simulink model "DFADAS2_SenFus_v1_201204RC_training_210115"  (R2018b)
settings: Solver=FixedStepDiscrete  StartTime=0.0  StopTime=inf  FixedStep=0.002  RelTol=1e-3  EnableMultiTasking=on
PreLoadFcn:
  | RTWConfigurationCB('preloadfcn', bdroot);
libraries: canmsglib x108, simulink x48, canfdmsglib x12
(part 15 of 28)

== system DFADAS2_SenFus_v1_201204RC_training_210115/Signal Input (Input)/Signal Input (50ms) (Input50)/Front Right Radar(S3) Objects Information (FRRdr)/S0 Data Frame Read/Enabled Subsystem/M2ObjInfo ==
  msg : Inport
  MValue : Inport  Port=2
  RemainderCnt : Inport  Port=3
  obj_num : Inport  Port=4
  Add3 : Sum
  Bus Creator1 : BusCreator  Inputs=24
  Bus Creator2 : BusCreator  Inputs=24
  Constant : Constant  Value=5
  Data Type Conversion{,1..3} (4 alike) : DataTypeConversion  OutDataTypeStr=uint16
  Data Type Conversion5 : DataTypeConversion  OutDataTypeStr=int16
  Demux : Demux  Outputs=24
  Demux1 : Demux  Outputs=24
  If : If  NumInputs=3  IfExpression=u1 == 1  ElseIfExpressions=u2 == 0 & u3 == 1  ShowElse=off
  If Action Subsystem1 : Subsystem  TreatAsAtomicUnit=on
  If Action Subsystem2 : Subsystem  TreatAsAtomicUnit=on
  MValueSel : Constant  Value=2
  Memory1 : Memory  InheritSampleTime=on
  Memory3 : Memory  InheritSampleTime=on
  Merge : Merge
  Merge1 : Merge
  Relational Operator : RelationalOperator  Operator===  OutDataTypeStr=boolean  RndMeth=Simplest
  Relational Operator1 : RelationalOperator  Operator=>  OutDataTypeStr=boolean  RndMeth=Simplest
  Subsystem1 : Subsystem
  Subtract : Sum  Inputs=+-
  M20ObjInfo : Outport
  M21ObjInfo : Outport  Port=2
  wires:
  msg/1 -> If Action Subsystem1/1(msg)
  MValue/1 -> Relational Operator/2
  Subsystem1/1(Out) -> Add3/2
  Add3/1 -> Memory3/1, Data Type Conversion2/1  "MValueSim"
  Data Type Conversion/1 -> Add3/1
  If/1 -> If Action Subsystem1/Action
  If/2 -> If Action Subsystem2/Action
  Relational Operator/1 -> Data Type Conversion/1, Data Type Conversion1/1
  If Action Subsystem1/1(M20ObjInfo) -> Merge/1
  If Action Subsystem2/1(ZeroObjInfo0) -> Merge/2
  MValueSel/1 -> If Action Subsystem1/2("MValueSel "), Relational Operator/1
  If Action Subsystem2/2(ZeroObjInfo1) -> Merge1/2
  If Action Subsystem1/2(M21ObjInfo) -> Merge1/1
  Data Type Conversion1/1 -> If/1
  Data Type Conversion2/1 -> If/2
  Data Type Conversion3/1 -> If/3
  Merge/1 -> Demux/1
  Bus Creator1/1 -> M20ObjInfo/1  "Obj5Info"
  Demux/24 -> Bus Creator1/24  "YVelocityStd_S0_005"
  Demux/10 -> Bus Creator1/10  "Width_S0_005"
  Demux/13 -> Bus Creator1/13  "ExistenceProb_S0_005"
  Demux/17 -> Bus Creator1/17  "ReferencePoint_S0_005"
  Demux/22 -> Bus Creator1/22  "YAccStd_S0_005"
  Demux/7 -> Bus Creator1/7  "YVelocity_S0_005"
  Demux/20 -> Bus Creator1/20  "XPosStd_S0_005"
  Demux/18 -> Bus Creator1/18  "Height_S0_005"
  Demux/12 -> Bus Creator1/12  "Orientation_S0_005"
  Demux/9 -> Bus Creator1/9  "YAcc_S0_005"
  Demux/14 -> Bus Creator1/14  "MovingState_S0_005"
  Demux/5 -> Bus Creator1/5  "YPos_S0_005"
  Demux/23 -> Bus Creator1/23  "YPosStd_S0_005"
  Demux/3 -> Bus Creator1/3  "ObjMeasured_S0_005"
  Demux/16 -> Bus Creator1/16  "ClassHighestProb_S0_005"
  Demux/21 -> Bus Creator1/21  "XVelocityStd_S0_005"
  Demux/4 -> Bus Creator1/4  "XPos_S0_005"
  Demux/19 -> Bus Creator1/19  "XAccStd_S0_005"
  Demux/8 -> Bus Creator1/8  "XAcc_S0_005"
  Demux/2 -> Bus Creator1/2  "ObjInit_S0_005"
  Demux/11 -> Bus Creator1/11  "Length_S0_005"
  Demux/15 -> Bus Creator1/15  "ClassHighest_S0_005"
  Demux/1 -> Bus Creator1/1  "Id_S0_005"
  Demux/6 -> Bus Creator1/6  "XVelocity_S0_005"
  Demux1/1 -> Bus Creator2/1  "Id_S0_006"
  Demux1/6 -> Bus Creator2/6  "XVelocity_S0_006"
  Demux1/2 -> Bus Creator2/2  "ObjInit_S0_006"
  Demux1/3 -> Bus Creator2/3  "ObjMeasured_S0_006"
  Demux1/5 -> Bus Creator2/5  "YPos_S0_006"
  Demux1/16 -> Bus Creator2/16  "ClassHighestProb_S0_006"
  Demux1/4 -> Bus Creator2/4  "XPos_S0_006"
  Demux1/10 -> Bus Creator2/10  "Width_S0_006"
  Demux1/11 -> Bus Creator2/11  "Length_S0_006"
  Demux1/24 -> Bus Creator2/24  "YVelocityStd_S0_006"
  Demux1/9 -> Bus Creator2/9  "YAcc_S0_006"
  Demux1/13 -> Bus Creator2/13  "ExistenceProb_S0_006"
  Demux1/20 -> Bus Creator2/20  "XPosStd_S0_006"
  Demux1/14 -> Bus Creator2/14  "MovingState_S0_006"
  Demux1/7 -> Bus Creator2/7  "YVelocity_S0_006"
  Demux1/15 -> Bus Creator2/15  "ClassHighest_S0_006"
  Demux1/18 -> Bus Creator2/18  "Height_S0_006"
  Demux1/19 -> Bus Creator2/19  "XAccStd_S0_006"
  Demux1/21 -> Bus Creator2/21  "XVelocityStd_S0_006"
  Demux1/8 -> Bus Creator2/8  "XAcc_S0_006"
  Demux1/23 -> Bus Creator2/23  "YPosStd_S0_006"
  Demux1/22 -> Bus Creator2/22  "YAccStd_S0_006"
  Demux1/17 -> Bus Creator2/17  "ReferencePoint_S0_006"
  Demux1/12 -> Bus Creator2/12  "Orientation_S0_006"
  Merge1/1 -> Demux1/1
  Bus Creator2/1 -> M21ObjInfo/1  "Obj6Info"
  Relational Operator1/1 -> If Action Subsystem1/3("obj_count_trorfa ")
  Constant/1 -> Relational Operator1/2
  obj_num/1 -> Relational Operator1/1
  Subtract/1 -> Subsystem1/1(const)
  RemainderCnt/1 -> Data Type Conversion5/1, Data Type Conversion3/1
  Memory1/1 -> Subtract/2
  Data Type Conversion5/1 -> Subtract/1, Memory1/1
  Memory3/1 -> Subsystem1/3(In)

== system DFADAS2_SenFus_v1_201204RC_training_210115/Signal Input (Input)/Signal Input (50ms) (Input50)/Front Right Radar(S3) Objects Information (FRRdr)/S0 Data Frame Read/Enabled Subsystem/M3ObjInfo ==
  msg : Inport
  MValue : Inport  Port=2
  RemainderCnt : Inport  Port=3
  obj_num : Inport  Port=4
  Add3 : Sum
  Bus Creator1 : BusCreator  Inputs=24
  Bus Creator2 : BusCreator  Inputs=24
  Constant : Constant  Value=7
  Data Type Conversion{,1..3} (4 alike) : DataTypeConversion  OutDataTypeStr=uint16
  Data Type Conversion5 : DataTypeConversion  OutDataTypeStr=int16
  Demux : Demux  Outputs=24
  Demux1 : Demux  Outputs=24
  If : If  NumInputs=3  IfExpression=u1 == 1  ElseIfExpressions=u2 == 0 & u3 == 1  ShowElse=off
  If Action Subsystem1 : Subsystem  TreatAsAtomicUnit=on
  If Action Subsystem2 : Subsystem  TreatAsAtomicUnit=on
  MValueSel : Constant  Value=3
  Memory1 : Memory  InheritSampleTime=on
  Memory3 : Memory  InheritSampleTime=on
  Merge : Merge
  Merge1 : Merge
  Relational Operator : RelationalOperator  Operator===  OutDataTypeStr=boolean  RndMeth=Simplest
  Relational Operator1 : RelationalOperator  Operator=>  OutDataTypeStr=boolean  RndMeth=Simplest
  Subsystem1 : Subsystem
  Subtract : Sum  Inputs=+-
  M30ObjInfo : Outport
  M31ObjInfo : Outport  Port=2
  wires:
  Bus Creator2/1 -> M31ObjInfo/1  "Obj8Info"
  Merge1/1 -> Demux1/1
  Demux1/12 -> Bus Creator2/12  "Orientation_S0_008"
  Demux1/17 -> Bus Creator2/17  "ReferencePoint_S0_008"
  Demux1/22 -> Bus Creator2/22  "YAccStd_S0_008"
  Demux1/23 -> Bus Creator2/23  "YPosStd_S0_008"
  Demux1/8 -> Bus Creator2/8  "XAcc_S0_008"
  Demux1/21 -> Bus Creator2/21  "XVelocityStd_S0_008"
  Demux1/19 -> Bus Creator2/19  "XAccStd_S0_008"
  Demux1/18 -> Bus Creator2/18  "Height_S0_008"
  Demux1/15 -> Bus Creator2/15  "ClassHighest_S0_008"
  Demux1/7 -> Bus Creator2/7  "YVelocity_S0_008"
  Demux1/14 -> Bus Creator2/14  "MovingState_S0_008"
  Demux1/20 -> Bus Creator2/20  "XPosStd_S0_008"
  Demux1/13 -> Bus Creator2/13  "ExistenceProb_S0_008"
  Demux1/9 -> Bus Creator2/9  "YAcc_S0_008"
  Demux1/24 -> Bus Creator2/24  "YVelocityStd_S0_008"
  Demux1/11 -> Bus Creator2/11  "Length_S0_008"
  Demux1/10 -> Bus Creator2/10  "Width_S0_008"
  Demux1/4 -> Bus Creator2/4  "XPos_S0_008"
  Demux1/16 -> Bus Creator2/16  "ClassHighestProb_S0_008"
  Demux1/5 -> Bus Creator2/5  "YPos_S0_008"
  Demux1/3 -> Bus Creator2/3  "ObjMeasured_S0_008"
  Demux1/2 -> Bus Creator2/2  "ObjInit_S0_008"
  Demux1/6 -> Bus Creator2/6  "XVelocity_S0_008"
  Demux1/1 -> Bus Creator2/1  "Id_S0_008"
  Demux/6 -> Bus Creator1/6  "XVelocity_S0_007"
  Demux/1 -> Bus Creator1/1  "Id_S0_007"
  Demux/15 -> Bus Creator1/15  "ClassHighest_S0_007"
  Demux/11 -> Bus Creator1/11  "Length_S0_007"
  Demux/2 -> Bus Creator1/2  "ObjInit_S0_007"
  Demux/8 -> Bus Creator1/8  "XAcc_S0_007"
  Demux/19 -> Bus Creator1/19  "XAccStd_S0_007"
  Demux/4 -> Bus Creator1/4  "XPos_S0_007"
  Demux/21 -> Bus Creator1/21  "XVelocityStd_S0_007"
  Demux/16 -> Bus Creator1/16  "ClassHighestProb_S0_007"
  Demux/3 -> Bus Creator1/3  "ObjMeasured_S0_007"
  Demux/23 -> Bus Creator1/23  "YPosStd_S0_007"
  Demux/5 -> Bus Creator1/5  "YPos_S0_007"
  Demux/14 -> Bus Creator1/14  "MovingState_S0_007"
  Demux/9 -> Bus Creator1/9  "YAcc_S0_007"
  Demux/12 -> Bus Creator1/12  "Orientation_S0_007"
  Demux/18 -> Bus Creator1/18  "Height_S0_007"
  Demux/20 -> Bus Creator1/20  "XPosStd_S0_007"
  Demux/7 -> Bus Creator1/7  "YVelocity_S0_007"
  Demux/22 -> Bus Creator1/22  "YAccStd_S0_007"
  Demux/17 -> Bus Creator1/17  "ReferencePoint_S0_007"
  Demux/13 -> Bus Creator1/13  "ExistenceProb_S0_007"
  Demux/10 -> Bus Creator1/10  "Width_S0_007"
  Demux/24 -> Bus Creator1/24  "YVelocityStd_S0_007"
  Bus Creator1/1 -> M30ObjInfo/1  "Obj7Info"
  Merge/1 -> Demux/1
  Data Type Conversion3/1 -> If/3
  Data Type Conversion2/1 -> If/2
  Data Type Conversion1/1 -> If/1
  If Action Subsystem1/2(M31ObjInfo) -> Merge1/1
  If Action Subsystem2/2(ZeroObjInfo1) -> Merge1/2
  MValueSel/1 -> Relational Operator/1, If Action Subsystem1/2("MValueSel ")
  If Action Subsystem2/1(ZeroObjInfo0) -> Merge/2
  If Action Subsystem1/1(M30ObjInfo) -> Merge/1
  Relational Operator/1 -> Data Type Conversion1/1, Data Type Conversion/1
  If/2 -> If Action Subsystem2/Action
  If/1 -> If Action Subsystem1/Action
  Data Type Conversion/1 -> Add3/1
  Add3/1 -> Memory3/1, Data Type Conversion2/1  "MValueSim"
  Subsystem1/1(Out) -> Add3/2
  MValue/1 -> Relational Operator/2
  msg/1 -> If Action Subsystem1/1(msg)
  Relational Operator1/1 -> If Action Subsystem1/3(obj_num)
  obj_num/1 -> Relational Operator1/1
  Constant/1 -> Relational Operator1/2
  Subtract/1 -> Subsystem1/1(const)
  RemainderCnt/1 -> Data Type Conversion5/1, Data Type Conversion3/1
  Memory1/1 -> Subtract/2
  Data Type Conversion5/1 -> Subtract/1, Memory1/1
  Memory3/1 -> Subsystem1/3(In)

== system DFADAS2_SenFus_v1_201204RC_training_210115/Signal Input (Input)/Signal Input (50ms) (Input50)/Front Right Radar(S3) Objects Information (FRRdr)/S0 Data Frame Read/Enabled Subsystem/M4ObjInfo1 ==
  msg : Inport
  MValue : Inport  Port=2
  RemainderCnt : Inport  Port=3
  obj_num : Inport  Port=4
  Add3 : Sum
  Bus Creator1 : BusCreator  Inputs=24
  Bus Creator2 : BusCreator  Inputs=24
  Constant : Constant  Value=9
  Data Type Conversion{,1..3} (4 alike) : DataTypeConversion  OutDataTypeStr=uint16
  Data Type Conversion5 : DataTypeConversion  OutDataTypeStr=int16
  Demux : Demux  Outputs=24
  Demux1 : Demux  Outputs=24
  If : If  NumInputs=3  IfExpression=u1 == 1  ElseIfExpressions=u2 == 0 & u3 == 1  ShowElse=off
  If Action Subsystem1 : Subsystem  TreatAsAtomicUnit=on
  If Action Subsystem2 : Subsystem  TreatAsAtomicUnit=on
  MValueSel : Constant  Value=4
  Memory1 : Memory  InheritSampleTime=on
  Memory2 : Memory  InheritSampleTime=on
  Merge : Merge
  Merge1 : Merge
  Relational Operator : RelationalOperator  Operator===  OutDataTypeStr=boolean  RndMeth=Simplest
  Relational Operator1 : RelationalOperator  Operator=>  OutDataTypeStr=boolean  RndMeth=Simplest
  Subsystem1 : Subsystem
  Subtract : Sum  Inputs=+-
  M40ObjInfo : Outport
  M41ObjInfo : Outport  Port=2
  wires:
  msg/1 -> If Action Subsystem1/1(msg)
  MValue/1 -> Relational Operator/2
  Add3/1 -> Memory2/1, Data Type Conversion2/1  "MValueSim"
  Data Type Conversion/1 -> Add3/1
  If/1 -> If Action Subsystem1/Action
  If/2 -> If Action Subsystem2/Action
  Relational Operator/1 -> Data Type Conversion/1, Data Type Conversion1/1
  If Action Subsystem1/1(M40ObjInfo) -> Merge/1
  If Action Subsystem2/1(ZeroObjInfo0) -> Merge/2
  MValueSel/1 -> If Action Subsystem1/2("MValueSel "), Relational Operator/1
  If Action Subsystem2/2(ZeroObjInfo1) -> Merge1/2
  If Action Subsystem1/2(M41ObjInfo) -> Merge1/1
  Data Type Conversion1/1 -> If/1
  Data Type Conversion2/1 -> If/2
  Data Type Conversion3/1 -> If/3
  Merge/1 -> Demux/1
  Bus Creator1/1 -> M40ObjInfo/1  "Obj9Info"
  Demux/24 -> Bus Creator1/24  "YVelocityStd_S0_009"
  Demux/10 -> Bus Creator1/10  "Width_S0_009"
  Demux/13 -> Bus Creator1/13  "ExistenceProb_S0_009"
  Demux/17 -> Bus Creator1/17  "ReferencePoint_S0_009"
  Demux/22 -> Bus Creator1/22  "YAccStd_S0_009"
  Demux/7 -> Bus Creator1/7  "YVelocity_S0_009"
  Demux/20 -> Bus Creator1/20  "XPosStd_S0_009"
  Demux/18 -> Bus Creator1/18  "Height_S0_009"
  Demux/12 -> Bus Creator1/12  "Orientation_S0_009"
  Demux/9 -> Bus Creator1/9  "YAcc_S0_009"
  Demux/14 -> Bus Creator1/14  "MovingState_S0_009"
  Demux/5 -> Bus Creator1/5  "YPos_S0_009"
  Demux/23 -> Bus Creator1/23  "YPosStd_S0_009"
  Demux/3 -> Bus Creator1/3  "ObjMeasured_S0_009"
  Demux/16 -> Bus Creator1/16  "ClassHighestProb_S0_009"
  Demux/21 -> Bus Creator1/21  "XVelocityStd_S0_009"
  Demux/4 -> Bus Creator1/4  "XPos_S0_009"
  Demux/19 -> Bus Creator1/19  "XAccStd_S0_009"
  Demux/8 -> Bus Creator1/8  "XAcc_S0_009"
  Demux/2 -> Bus Creator1/2  "ObjInit_S0_009"
  Demux/11 -> Bus Creator1/11  "Length_S0_009"
  Demux/15 -> Bus Creator1/15  "ClassHighest_S0_009"
  Demux/1 -> Bus Creator1/1  "Id_S0_009"
  Demux/6 -> Bus Creator1/6  "XVelocity_S0_009"
  Demux1/1 -> Bus Creator2/1  "Id_S0_010"
  Demux1/6 -> Bus Creator2/6  "XVelocity_S0_010"
  Demux1/2 -> Bus Creator2/2  "ObjInit_S0_010"
  Demux1/3 -> Bus Creator2/3  "ObjMeasured_S0_010"
  Demux1/5 -> Bus Creator2/5  "YPos_S0_010"
  Demux1/16 -> Bus Creator2/16  "ClassHighestProb_S0_010"
  Demux1/4 -> Bus Creator2/4  "XPos_S0_010"
  Demux1/10 -> Bus Creator2/10  "Width_S0_010"
  Demux1/11 -> Bus Creator2/11  "Length_S0_010"
  Demux1/24 -> Bus Creator2/24  "YVelocityStd_S0_010"
  Demux1/9 -> Bus Creator2/9  "YAcc_S0_010"
  Demux1/13 -> Bus Creator2/13  "ExistenceProb_S0_010"
  Demux1/20 -> Bus Creator2/20  "XPosStd_S0_010"
  Demux1/14 -> Bus Creator2/14  "MovingState_S0_010"
  Demux1/7 -> Bus Creator2/7  "YVelocity_S0_010"
  Demux1/15 -> Bus Creator2/15  "ClassHighest_S0_010"
  Demux1/18 -> Bus Creator2/18  "Height_S0_010"
  Demux1/19 -> Bus Creator2/19  "XAccStd_S0_010"
  Demux1/21 -> Bus Creator2/21  "XVelocityStd_S0_010"
  Demux1/8 -> Bus Creator2/8  "XAcc_S0_010"
  Demux1/23 -> Bus Creator2/23  "YPosStd_S0_010"
  Demux1/22 -> Bus Creator2/22  "YAccStd_S0_010"
  Demux1/17 -> Bus Creator2/17  "ReferencePoint_S0_010"
  Demux1/12 -> Bus Creator2/12  "Orientation_S0_010"
  Merge1/1 -> Demux1/1
  Bus Creator2/1 -> M41ObjInfo/1  "Obj10Info"
  Relational Operator1/1 -> If Action Subsystem1/3("obj_num ")
  obj_num/1 -> Relational Operator1/1
  Constant/1 -> Relational Operator1/2
  Subtract/1 -> Subsystem1/1(const)
  RemainderCnt/1 -> Data Type Conversion5/1, Data Type Conversion3/1
  Memory1/1 -> Subtract/2
  Data Type Conversion5/1 -> Subtract/1, Memory1/1
  Memory2/1 -> Subsystem1/3(In)
  Subsystem1/1(Out) -> Add3/2

== system DFADAS2_SenFus_v1_201204RC_training_210115/Signal Input (Input)/Signal Input (50ms) (Input50)/Front Right Radar(S3) Objects Information (FRRdr)/S0 Data Frame Read/Enabled Subsystem/Unpack ==
  Msg : Inport
  RemainderCnt : Inport  Port=2
  Add : Sum
  Bus Selector : BusSelector  Commented=on  OutputSignals=Obj1Info.Id_S0_001
  Constant : Constant  Value=0
  If : If  IfExpression=u1>0  ElseIfExpressions=u1==0
  If Action Subsystem : Subsystem  TreatAsAtomicUnit=on
  If Action Subsystem1 : Subsystem  TreatAsAtomicUnit=on
  Merge : Merge
  Scope : Scope  Commented=on
  MsgOut : Outport
  MValue : Outport  Port=2
  wires:
  If/2 -> If Action Subsystem1/Action
  Msg/1 -> If Action Subsystem/1(msg)
  If/1 -> If Action Subsystem/Action
  If Action Subsystem/1(FRRdrObjInfo) -> Bus Selector/1, MsgOut/1
  If Action Subsystem/2(MValue) -> Add/1
  If Action Subsystem1/1(DflMValue) -> Merge/2
  Add/1 -> Merge/1
  Bus Selector/1 -> Scope/1  "<Id_S0_001>"
  Constant/1 -> Add/2
  Merge/1 -> MValue/1
  RemainderCnt/1 -> If/1

== system DFADAS2_SenFus_v1_201204RC_training_210115/Signal Input (Input)/Signal Input (50ms) (Input50)/Front Right Radar(S3) Objects Information (FRRdr)/S0 Data Frame Read/Subsystem/M0ObjInfo ==
  Bus Creator1 : BusCreator  Inputs=24
  Bus Creator2 : BusCreator  Inputs=24
  Constant : Constant  Value=[0 0 0 0 0 0 0 0 0 0 0 0 0 0 0 0 0 0 0 0 0 0 0 0 ]
  Constant1 : Constant  Value=[0 0 0 0 0 0 0 0 0 0 0 0 0 0 0 0 0 0 0 0 0 0 0 0 ]
  Demux : Demux  Outputs=24
  Demux1 : Demux  Outputs=24
  M00ObjInfo : Outport
  M01ObjInfo : Outport  Port=2
  wires:
  Demux1/23 -> Bus Creator2/23  "YPosStd_S0_002"
  Demux1/17 -> Bus Creator2/17  "ReferencePoint_S0_002"
  Demux/1 -> Bus Creator1/1  "Id_S0_001"
  Demux1/10 -> Bus Creator2/10  "Width_S0_002"
  Demux1/22 -> Bus Creator2/22  "YAccStd_S0_002"
  Demux1/19 -> Bus Creator2/19  "XAccStd_S0_002"
  Demux/20 -> Bus Creator1/20  "XPosStd_S0_001"
  Demux/5 -> Bus Creator1/5  "YPos_S0_001"
  Demux1/8 -> Bus Creator2/8  "XAcc_S0_002"
  Demux1/15 -> Bus Creator2/15  "ClassHighest_S0_002"
  Demux/21 -> Bus Creator1/21  "XVelocityStd_S0_001"
  Constant1/1 -> Demux1/1
  Demux1/1 -> Bus Creator2/1  "Id_S0_002"
  Demux1/9 -> Bus Creator2/9  "YAcc_S0_002"
  Demux1/14 -> Bus Creator2/14  "MovingState_S0_002"
  Demux1/5 -> Bus Creator2/5  "YPos_S0_002"
  Demux1/16 -> Bus Creator2/16  "ClassHighestProb_S0_002"
  Demux1/11 -> Bus Creator2/11  "Length_S0_002"
  Demux/24 -> Bus Creator1/24  "YVelocityStd_S0_001"
  Demux/19 -> Bus Creator1/19  "XAccStd_S0_001"
  Demux/16 -> Bus Creator1/16  "ClassHighestProb_S0_001"
  Demux/13 -> Bus Creator1/13  "ExistenceProb_S0_001"
  Demux/15 -> Bus Creator1/15  "ClassHighest_S0_001"
  Demux/18 -> Bus Creator1/18  "Height_S0_001"
  Demux/4 -> Bus Creator1/4  "XPos_S0_001"
  Demux/2 -> Bus Creator1/2  "ObjInit_S0_001"
  Demux/7 -> Bus Creator1/7  "YVelocity_S0_001"
  Demux1/13 -> Bus Creator2/13  "ExistenceProb_S0_002"
  Demux1/7 -> Bus Creator2/7  "YVelocity_S0_002"
  Demux/6 -> Bus Creator1/6  "XVelocity_S0_001"
  Demux1/12 -> Bus Creator2/12  "Orientation_S0_002"
  Demux/14 -> Bus Creator1/14  "MovingState_S0_001"
  Demux/11 -> Bus Creator1/11  "Length_S0_001"
  Demux/3 -> Bus Creator1/3  "ObjMeasured_S0_001"
  Demux1/24 -> Bus Creator2/24  "YVelocityStd_S0_002"
  Demux/9 -> Bus Creator1/9  "YAcc_S0_001"
  Demux1/4 -> Bus Creator2/4  "XPos_S0_002"
  Demux/23 -> Bus Creator1/23  "YPosStd_S0_001"
  Demux1/21 -> Bus Creator2/21  "XVelocityStd_S0_002"
  Demux1/20 -> Bus Creator2/20  "XPosStd_S0_002"
  Bus Creator2/1 -> M01ObjInfo/1  "Obj2Info"
  Demux/17 -> Bus Creator1/17  "ReferencePoint_S0_001"
  Bus Creator1/1 -> M00ObjInfo/1
  Demux1/2 -> Bus Creator2/2  "ObjInit_S0_002"
  Demux/10 -> Bus Creator1/10  "Width_S0_001"
  Constant/1 -> Demux/1
  Demux/8 -> Bus Creator1/8  "XAcc_S0_001"
  Demux/12 -> Bus Creator1/12  "Orientation_S0_001"
  Demux1/18 -> Bus Creator2/18  "Height_S0_002"
  Demux/22 -> Bus Creator1/22  "YAccStd_S0_001"
  Demux1/3 -> Bus Creator2/3  "ObjMeasured_S0_002"
  Demux1/6 -> Bus Creator2/6  "XVelocity_S0_002"

== system DFADAS2_SenFus_v1_201204RC_training_210115/Signal Input (Input)/Signal Input (50ms) (Input50)/Front Right Radar(S3) Objects Information (FRRdr)/S0 Data Frame Read/Subsystem/M1ObjInfo1 ==
  Bus Creator1 : BusCreator  Inputs=24
  Bus Creator2 : BusCreator  Inputs=24
  Constant : Constant  Value=[0 0 0 0 0 0 0 0 0 0 0 0 0 0 0 0 0 0 0 0 0 0 0 0 ]
  Constant1 : Constant  Value=[0 0 0 0 0 0 0 0 0 0 0 0 0 0 0 0 0 0 0 0 0 0 0 0 ]
  Demux : Demux  Outputs=24
  Demux1 : Demux  Outputs=24
  M10ObjInfo : Outport
  M11ObjInfo : Outport  Port=2
  wires:
  Bus Creator2/1 -> M11ObjInfo/1  "Obj4Info"
  Demux1/12 -> Bus Creator2/12  "Orientation_S0_004"
  Demux1/17 -> Bus Creator2/17  "ReferencePoint_S0_004"
  Demux1/22 -> Bus Creator2/22  "YAccStd_S0_004"
  Demux1/23 -> Bus Creator2/23  "YPosStd_S0_004"
  Demux1/8 -> Bus Creator2/8  "XAcc_S0_004"
  Demux1/21 -> Bus Creator2/21  "XVelocityStd_S0_004"
  Demux1/19 -> Bus Creator2/19  "XAccStd_S0_004"
  Demux1/18 -> Bus Creator2/18  "Height_S0_004"
  Demux1/15 -> Bus Creator2/15  "ClassHighest_S0_004"
  Demux1/7 -> Bus Creator2/7  "YVelocity_S0_004"
  Demux1/14 -> Bus Creator2/14  "MovingState_S0_004"
  Demux1/20 -> Bus Creator2/20  "XPosStd_S0_004"
  Demux1/13 -> Bus Creator2/13  "ExistenceProb_S0_004"
  Demux1/9 -> Bus Creator2/9  "YAcc_S0_004"
  Demux1/24 -> Bus Creator2/24  "YVelocityStd_S0_004"
  Demux1/11 -> Bus Creator2/11  "Length_S0_004"
  Demux1/10 -> Bus Creator2/10  "Width_S0_004"
  Demux1/4 -> Bus Creator2/4  "XPos_S0_004"
  Demux1/16 -> Bus Creator2/16  "ClassHighestProb_S0_004"
  Demux1/5 -> Bus Creator2/5  "YPos_S0_004"
  Demux1/3 -> Bus Creator2/3  "ObjMeasured_S0_004"
  Demux1/2 -> Bus Creator2/2  "ObjInit_S0_004"
  Demux1/6 -> Bus Creator2/6  "XVelocity_S0_004"
  Demux1/1 -> Bus Creator2/1  "Id_S0_004"
  Demux/6 -> Bus Creator1/6  "XVelocity_S0_003"
  Demux/1 -> Bus Creator1/1  "Id_S0_003"
  Demux/15 -> Bus Creator1/15  "ClassHighest_S0_003"
  Demux/11 -> Bus Creator1/11  "Length_S0_003"
  Demux/2 -> Bus Creator1/2  "ObjInit_S0_003"
  Demux/8 -> Bus Creator1/8  "XAcc_S0_003"
  Demux/19 -> Bus Creator1/19  "XAccStd_S0_003"
  Demux/4 -> Bus Creator1/4  "XPos_S0_003"
  Demux/21 -> Bus Creator1/21  "XVelocityStd_S0_003"
  Demux/16 -> Bus Creator1/16  "ClassHighestProb_S0_003"
  Demux/3 -> Bus Creator1/3  "ObjMeasured_S0_003"
  Demux/23 -> Bus Creator1/23  "YPosStd_S0_003"
  Demux/5 -> Bus Creator1/5  "YPos_S0_003"
  Demux/14 -> Bus Creator1/14  "MovingState_S0_003"
  Demux/9 -> Bus Creator1/9  "YAcc_S0_003"
  Demux/12 -> Bus Creator1/12  "Orientation_S0_003"
  Demux/18 -> Bus Creator1/18  "Height_S0_003"
  Demux/20 -> Bus Creator1/20  "XPosStd_S0_003"
  Demux/7 -> Bus Creator1/7  "YVelocity_S0_003"
  Demux/22 -> Bus Creator1/22  "YAccStd_S0_003"
  Demux/17 -> Bus Creator1/17  "ReferencePoint_S0_003"
  Demux/13 -> Bus Creator1/13  "ExistenceProb_S0_003"
  Demux/10 -> Bus Creator1/10  "Width_S0_003"
  Demux/24 -> Bus Creator1/24  "YVelocityStd_S0_003"
  Bus Creator1/1 -> M10ObjInfo/1  "Obj3Info"
  Constant/1 -> Demux/1
  Constant1/1 -> Demux1/1

== system DFADAS2_SenFus_v1_201204RC_training_210115/Signal Input (Input)/Signal Input (50ms) (Input50)/Front Right Radar(S3) Objects Information (FRRdr)/S0 Data Frame Read/Subsystem/M2ObjInfo ==
  Bus Creator1 : BusCreator  Inputs=24
  Bus Creator2 : BusCreator  Inputs=24
  Constant : Constant  Value=[0 0 0 0 0 0 0 0 0 0 0 0 0 0 0 0 0 0 0 0 0 0 0 0 ]
  Constant1 : Constant  Value=[0 0 0 0 0 0 0 0 0 0 0 0 0 0 0 0 0 0 0 0 0 0 0 0 ]
  Demux : Demux  Outputs=24
  Demux1 : Demux  Outputs=24
  M20ObjInfo : Outport
  M21ObjInfo : Outport  Port=2
  wires:
  Constant/1 -> Demux/1
  Bus Creator1/1 -> M20ObjInfo/1  "Obj5Info"
  Demux/24 -> Bus Creator1/24  "YVelocityStd_S0_005"
  Demux/10 -> Bus Creator1/10  "Width_S0_005"
  Demux/13 -> Bus Creator1/13  "ExistenceProb_S0_005"
  Demux/17 -> Bus Creator1/17  "ReferencePoint_S0_005"
  Demux/22 -> Bus Creator1/22  "YAccStd_S0_005"
  Demux/7 -> Bus Creator1/7  "YVelocity_S0_005"
  Demux/20 -> Bus Creator1/20  "XPosStd_S0_005"
  Demux/18 -> Bus Creator1/18  "Height_S0_005"
  Demux/12 -> Bus Creator1/12  "Orientation_S0_005"
  Demux/9 -> Bus Creator1/9  "YAcc_S0_005"
  Demux/14 -> Bus Creator1/14  "MovingState_S0_005"
  Demux/5 -> Bus Creator1/5  "YPos_S0_005"
  Demux/23 -> Bus Creator1/23  "YPosStd_S0_005"
  Demux/3 -> Bus Creator1/3  "ObjMeasured_S0_005"
  Demux/16 -> Bus Creator1/16  "ClassHighestProb_S0_005"
  Demux/21 -> Bus Creator1/21  "XVelocityStd_S0_005"
  Demux/4 -> Bus Creator1/4  "XPos_S0_005"
  Demux/19 -> Bus Creator1/19  "XAccStd_S0_005"
  Demux/8 -> Bus Creator1/8  "XAcc_S0_005"
  Demux/2 -> Bus Creator1/2  "ObjInit_S0_005"
  Demux/11 -> Bus Creator1/11  "Length_S0_005"
  Demux/15 -> Bus Creator1/15  "ClassHighest_S0_005"
  Demux/1 -> Bus Creator1/1  "Id_S0_005"
  Demux/6 -> Bus Creator1/6  "XVelocity_S0_005"
  Demux1/1 -> Bus Creator2/1  "Id_S0_006"
  Demux1/6 -> Bus Creator2/6  "XVelocity_S0_006"
  Demux1/2 -> Bus Creator2/2  "ObjInit_S0_006"
  Demux1/3 -> Bus Creator2/3  "ObjMeasured_S0_006"
  Demux1/5 -> Bus Creator2/5  "YPos_S0_006"
  Demux1/16 -> Bus Creator2/16  "ClassHighestProb_S0_006"
  Demux1/4 -> Bus Creator2/4  "XPos_S0_006"
  Demux1/10 -> Bus Creator2/10  "Width_S0_006"
  Demux1/11 -> Bus Creator2/11  "Length_S0_006"
  Demux1/24 -> Bus Creator2/24  "YVelocityStd_S0_006"
  Demux1/9 -> Bus Creator2/9  "YAcc_S0_006"
  Demux1/13 -> Bus Creator2/13  "ExistenceProb_S0_006"
  Demux1/20 -> Bus Creator2/20  "XPosStd_S0_006"
  Demux1/14 -> Bus Creator2/14  "MovingState_S0_006"
  Demux1/7 -> Bus Creator2/7  "YVelocity_S0_006"
  Demux1/15 -> Bus Creator2/15  "ClassHighest_S0_006"
  Demux1/18 -> Bus Creator2/18  "Height_S0_006"
  Demux1/19 -> Bus Creator2/19  "XAccStd_S0_006"
  Demux1/21 -> Bus Creator2/21  "XVelocityStd_S0_006"
  Demux1/8 -> Bus Creator2/8  "XAcc_S0_006"
  Demux1/23 -> Bus Creator2/23  "YPosStd_S0_006"
  Demux1/22 -> Bus Creator2/22  "YAccStd_S0_006"
  Demux1/17 -> Bus Creator2/17  "ReferencePoint_S0_006"
  Demux1/12 -> Bus Creator2/12  "Orientation_S0_006"
  Bus Creator2/1 -> M21ObjInfo/1  "Obj6Info"
  Constant1/1 -> Demux1/1

== system DFADAS2_SenFus_v1_201204RC_training_210115/Signal Input (Input)/Signal Input (50ms) (Input50)/Front Right Radar(S3) Objects Information (FRRdr)/S0 Data Frame Read/Subsystem/M3ObjInfo ==
  Bus Creator1 : BusCreator  Inputs=24
  Bus Creator2 : BusCreator  Inputs=24
  Constant : Constant  Value=[0 0 0 0 0 0 0 0 0 0 0 0 0 0 0 0 0 0 0 0 0 0 0 0 ]
  Constant1 : Constant  Value=[0 0 0 0 0 0 0 0 0 0 0 0 0 0 0 0 0 0 0 0 0 0 0 0 ]
  Demux : Demux  Outputs=24
  Demux1 : Demux  Outputs=24
  M30ObjInfo : Outport
  M31ObjInfo : Outport  Port=2
  wires:
  Bus Creator2/1 -> M31ObjInfo/1  "Obj8Info"
  Demux1/12 -> Bus Creator2/12  "Orientation_S0_008"
  Demux1/17 -> Bus Creator2/17  "ReferencePoint_S0_008"
  Demux1/22 -> Bus Creator2/22  "YAccStd_S0_008"
  Demux1/23 -> Bus Creator2/23  "YPosStd_S0_008"
  Demux1/8 -> Bus Creator2/8  "XAcc_S0_008"
  Demux1/21 -> Bus Creator2/21  "XVelocityStd_S0_008"
  Demux1/19 -> Bus Creator2/19  "XAccStd_S0_008"
  Demux1/18 -> Bus Creator2/18  "Height_S0_008"
  Demux1/15 -> Bus Creator2/15  "ClassHighest_S0_008"
  Demux1/7 -> Bus Creator2/7  "YVelocity_S0_008"
  Demux1/14 -> Bus Creator2/14  "MovingState_S0_008"
  Demux1/20 -> Bus Creator2/20  "XPosStd_S0_008"
  Demux1/13 -> Bus Creator2/13  "ExistenceProb_S0_008"
  Demux1/9 -> Bus Creator2/9  "YAcc_S0_008"
  Demux1/24 -> Bus Creator2/24  "YVelocityStd_S0_008"
  Demux1/11 -> Bus Creator2/11  "Length_S0_008"
  Demux1/10 -> Bus Creator2/10  "Width_S0_008"
  Demux1/4 -> Bus Creator2/4  "XPos_S0_008"
  Demux1/16 -> Bus Creator2/16  "ClassHighestProb_S0_008"
  Demux1/5 -> Bus Creator2/5  "YPos_S0_008"
  Demux1/3 -> Bus Creator2/3  "ObjMeasured_S0_008"
  Demux1/2 -> Bus Creator2/2  "ObjInit_S0_008"
  Demux1/6 -> Bus Creator2/6  "XVelocity_S0_008"
  Demux1/1 -> Bus Creator2/1  "Id_S0_008"
  Demux/6 -> Bus Creator1/6  "XVelocity_S0_007"
  Demux/1 -> Bus Creator1/1  "Id_S0_007"
  Demux/15 -> Bus Creator1/15  "ClassHighest_S0_007"
  Demux/11 -> Bus Creator1/11  "Length_S0_007"
  Demux/2 -> Bus Creator1/2  "ObjInit_S0_007"
  Demux/8 -> Bus Creator1/8  "XAcc_S0_007"
  Demux/19 -> Bus Creator1/19  "XAccStd_S0_007"
  Demux/4 -> Bus Creator1/4  "XPos_S0_007"
  Demux/21 -> Bus Creator1/21  "XVelocityStd_S0_007"
  Demux/16 -> Bus Creator1/16  "ClassHighestProb_S0_007"
  Demux/3 -> Bus Creator1/3  "ObjMeasured_S0_007"
  Demux/23 -> Bus Creator1/23  "YPosStd_S0_007"
  Demux/5 -> Bus Creator1/5  "YPos_S0_007"
  Demux/14 -> Bus Creator1/14  "MovingState_S0_007"
  Demux/9 -> Bus Creator1/9  "YAcc_S0_007"
  Demux/12 -> Bus Creator1/12  "Orientation_S0_007"
  Demux/18 -> Bus Creator1/18  "Height_S0_007"
  Demux/20 -> Bus Creator1/20  "XPosStd_S0_007"
  Demux/7 -> Bus Creator1/7  "YVelocity_S0_007"
  Demux/22 -> Bus Creator1/22  "YAccStd_S0_007"
  Demux/17 -> Bus Creator1/17  "ReferencePoint_S0_007"
  Demux/13 -> Bus Creator1/13  "ExistenceProb_S0_007"
  Demux/10 -> Bus Creator1/10  "Width_S0_007"
  Demux/24 -> Bus Creator1/24  "YVelocityStd_S0_007"
  Bus Creator1/1 -> M30ObjInfo/1  "Obj7Info"
  Constant/1 -> Demux/1
  Constant1/1 -> Demux1/1

== system DFADAS2_SenFus_v1_201204RC_training_210115/Signal Input (Input)/Signal Input (50ms) (Input50)/Front Right Radar(S3) Objects Information (FRRdr)/S0 Data Frame Read/Subsystem/M4ObjInfo1 ==
  Bus Creator1 : BusCreator  Inputs=24
  Bus Creator2 : BusCreator  Inputs=24
  Constant : Constant  Value=[0 0 0 0 0 0 0 0 0 0 0 0 0 0 0 0 0 0 0 0 0 0 0 0 ]
  Constant1 : Constant  Value=[0 0 0 0 0 0 0 0 0 0 0 0 0 0 0 0 0 0 0 0 0 0 0 0 ]
  Demux : Demux  Outputs=24
  Demux1 : Demux  Outputs=24
  M40ObjInfo : Outport
  M41ObjInfo : Outport  Port=2
  wires:
  Bus Creator1/1 -> M40ObjInfo/1  "Obj9Info"
  Demux/24 -> Bus Creator1/24  "YVelocityStd_S0_009"
  Demux/10 -> Bus Creator1/10  "Width_S0_009"
  Demux/13 -> Bus Creator1/13  "ExistenceProb_S0_009"
  Demux/17 -> Bus Creator1/17  "ReferencePoint_S0_009"
  Demux/22 -> Bus Creator1/22  "YAccStd_S0_009"
  Demux/7 -> Bus Creator1/7  "YVelocity_S0_009"
  Demux/20 -> Bus Creator1/20  "XPosStd_S0_009"
  Demux/18 -> Bus Creator1/18  "Height_S0_009"
  Demux/12 -> Bus Creator1/12  "Orientation_S0_009"
  Demux/9 -> Bus Creator1/9  "YAcc_S0_009"
  Demux/14 -> Bus Creator1/14  "MovingState_S0_009"
  Demux/5 -> Bus Creator1/5  "YPos_S0_009"
  Demux/23 -> Bus Creator1/23  "YPosStd_S0_009"
  Demux/3 -> Bus Creator1/3  "ObjMeasured_S0_009"
  Demux/16 -> Bus Creator1/16  "ClassHighestProb_S0_009"
  Demux/21 -> Bus Creator1/21  "XVelocityStd_S0_009"
  Demux/4 -> Bus Creator1/4  "XPos_S0_009"
  Demux/19 -> Bus Creator1/19  "XAccStd_S0_009"
  Demux/8 -> Bus Creator1/8  "XAcc_S0_009"
  Demux/2 -> Bus Creator1/2  "ObjInit_S0_009"
  Demux/11 -> Bus Creator1/11  "Length_S0_009"
  Demux/15 -> Bus Creator1/15  "ClassHighest_S0_009"
  Demux/1 -> Bus Creator1/1  "Id_S0_009"
  Demux/6 -> Bus Creator1/6  "XVelocity_S0_009"
  Demux1/1 -> Bus Creator2/1  "Id_S0_010"
  Demux1/6 -> Bus Creator2/6  "XVelocity_S0_010"
  Demux1/2 -> Bus Creator2/2  "ObjInit_S0_010"
  Demux1/3 -> Bus Creator2/3  "ObjMeasured_S0_010"
  Demux1/5 -> Bus Creator2/5  "YPos_S0_010"
  Demux1/16 -> Bus Creator2/16  "ClassHighestProb_S0_010"
  Demux1/4 -> Bus Creator2/4  "XPos_S0_010"
  Demux1/10 -> Bus Creator2/10  "Width_S0_010"
  Demux1/11 -> Bus Creator2/11  "Length_S0_010"
  Demux1/24 -> Bus Creator2/24  "YVelocityStd_S0_010"
  Demux1/9 -> Bus Creator2/9  "YAcc_S0_010"
  Demux1/13 -> Bus Creator2/13  "ExistenceProb_S0_010"
  Demux1/20 -> Bus Creator2/20  "XPosStd_S0_010"
  Demux1/14 -> Bus Creator2/14  "MovingState_S0_010"
  Demux1/7 -> Bus Creator2/7  "YVelocity_S0_010"
  Demux1/15 -> Bus Creator2/15  "ClassHighest_S0_010"
  Demux1/18 -> Bus Creator2/18  "Height_S0_010"
  Demux1/19 -> Bus Creator2/19  "XAccStd_S0_010"
  Demux1/21 -> Bus Creator2/21  "XVelocityStd_S0_010"
  Demux1/8 -> Bus Creator2/8  "XAcc_S0_010"
  Demux1/23 -> Bus Creator2/23  "YPosStd_S0_010"
  Demux1/22 -> Bus Creator2/22  "YAccStd_S0_010"
  Demux1/17 -> Bus Creator2/17  "ReferencePoint_S0_010"
  Demux1/12 -> Bus Creator2/12  "Orientation_S0_010"
  Bus Creator2/1 -> M41ObjInfo/1  "Obj10Info"
  Constant/1 -> Demux/1
  Constant1/1 -> Demux1/1

== system DFADAS2_SenFus_v1_201204RC_training_210115/Signal Input (Input)/Signal Input (50ms) (Input50)/Rear Left Radar(S0) Objects Information (RLRdr)/S0 Data Frame Read/Enabled Subsystem/M0ObjInfo ==
  msg : Inport
  MValue : Inport  Port=2
  RemainderCnt : Inport  Port=3
  obj_num : Inport  Port=4
  Add3 : Sum
  Bus Creator1 : BusCreator  Inputs=24
  Bus Creator2 : BusCreator  Inputs=24
  Constant : Constant
  Data Type Conversion{,1..3} (4 alike) : DataTypeConversion  OutDataTypeStr=uint16
  Data Type Conversion5 : DataTypeConversion  OutDataTypeStr=int16
  Demux : Demux  Outputs=24
  Demux1 : Demux  Outputs=24
  If : If  NumInputs=3  IfExpression=u1 == 1  ElseIfExpressions=u2 == 0&u3==1  ShowElse=off
  If Action Subsystem1 : Subsystem  TreatAsAtomicUnit=on
  If Action Subsystem2 : Subsystem  TreatAsAtomicUnit=on
  MValueSel : Constant  Value=0
  Memory2 : Memory  InheritSampleTime=on
  Memory3 : Memory  InheritSampleTime=on
  Merge : Merge
  Merge1 : Merge
  Relational Operator : RelationalOperator  Operator===  OutDataTypeStr=boolean  RndMeth=Simplest
  Relational Operator1 : RelationalOperator  Operator=>  OutDataTypeStr=boolean  RndMeth=Simplest
  Subsystem1 : Subsystem
  Subtract : Sum  Inputs=+-
  remainder_num : Constant  Value=0  OutDataTypeStr=uint16
  M00ObjInfo : Outport
  M01ObjInfo : Outport  Port=2
  wires:
  msg/1 -> If Action Subsystem1/1(msg)
  MValue/1 -> Relational Operator/2
  Add3/1 -> Memory3/1, Data Type Conversion2/1  "MValueSim"
  Data Type Conversion/1 -> Add3/1
  If/1 -> If Action Subsystem1/Action
  If/2 -> If Action Subsystem2/Action
  Relational Operator/1 -> Data Type Conversion/1, Data Type Conversion1/1
  If Action Subsystem1/1(M00ObjInfo) -> Merge/1
  If Action Subsystem2/1(ZeroObjInfo0) -> Merge/2
  MValueSel/1 -> If Action Subsystem1/2("MValueSel "), Relational Operator/1
  If Action Subsystem2/2(ZeroObjInfo1) -> Merge1/2
  If Action Subsystem1/2(M01ObjInfo) -> Merge1/1
  Merge/1 -> Demux/1
  Bus Creator1/1 -> M00ObjInfo/1
  Demux/24 -> Bus Creator1/24  "YVelocityStd_S0_001"
  Demux/10 -> Bus Creator1/10  "Width_S0_001"
  Demux/13 -> Bus Creator1/13  "ExistenceProb_S0_001"
  Demux/17 -> Bus Creator1/17  "ReferencePoint_S0_001"
  Demux/22 -> Bus Creator1/22  "YAccStd_S0_001"
  Demux/7 -> Bus Creator1/7  "YVelocity_S0_001"
  Demux/20 -> Bus Creator1/20  "XPosStd_S0_001"
  Demux/18 -> Bus Creator1/18  "Height_S0_001"
  Demux/12 -> Bus Creator1/12  "Orientation_S0_001"
  Demux/9 -> Bus Creator1/9  "YAcc_S0_001"
  Demux/14 -> Bus Creator1/14  "MovingState_S0_001"
  Demux/5 -> Bus Creator1/5  "YPos_S0_001"
  Demux/23 -> Bus Creator1/23  "YPosStd_S0_001"
  Demux/3 -> Bus Creator1/3  "ObjMeasured_S0_001"
  Demux/16 -> Bus Creator1/16  "ClassHighestProb_S0_001"
  Demux/21 -> Bus Creator1/21  "XVelocityStd_S0_001"
  Demux/4 -> Bus Creator1/4  "XPos_S0_001"
  Demux/19 -> Bus Creator1/19  "XAccStd_S0_001"
  Demux/8 -> Bus Creator1/8  "XAcc_S0_001"
  Demux/2 -> Bus Creator1/2  "ObjInit_S0_001"
  Demux/11 -> Bus Creator1/11  "Length_S0_001"
  Demux/15 -> Bus Creator1/15  "ClassHighest_S0_001"
  Demux/1 -> Bus Creator1/1  "Id_S0_001"
  Demux/6 -> Bus Creator1/6  "XVelocity_S0_001"
  Demux1/1 -> Bus Creator2/1  "Id_S0_002"
  Demux1/6 -> Bus Creator2/6  "XVelocity_S0_002"
  Demux1/2 -> Bus Creator2/2  "ObjInit_S0_002"
  Demux1/3 -> Bus Creator2/3  "ObjMeasured_S0_002"
  Demux1/5 -> Bus Creator2/5  "YPos_S0_002"
  Demux1/16 -> Bus Creator2/16  "ClassHighestProb_S0_002"
  Demux1/4 -> Bus Creator2/4  "XPos_S0_002"
  Demux1/10 -> Bus Creator2/10  "Width_S0_002"
  Demux1/11 -> Bus Creator2/11  "Length_S0_002"
  Demux1/24 -> Bus Creator2/24  "YVelocityStd_S0_002"
  Demux1/9 -> Bus Creator2/9  "YAcc_S0_002"
  Demux1/13 -> Bus Creator2/13  "ExistenceProb_S0_002"
  Demux1/20 -> Bus Creator2/20  "XPosStd_S0_002"
  Demux1/14 -> Bus Creator2/14  "MovingState_S0_002"
  Demux1/7 -> Bus Creator2/7  "YVelocity_S0_002"
  Demux1/15 -> Bus Creator2/15  "ClassHighest_S0_002"
  Demux1/18 -> Bus Creator2/18  "Height_S0_002"
  Demux1/19 -> Bus Creator2/19  "XAccStd_S0_002"
  Demux1/21 -> Bus Creator2/21  "XVelocityStd_S0_002"
  Demux1/8 -> Bus Creator2/8  "XAcc_S0_002"
  Demux1/23 -> Bus Creator2/23  "YPosStd_S0_002"
  Demux1/22 -> Bus Creator2/22  "YAccStd_S0_002"
  Demux1/17 -> Bus Creator2/17  "ReferencePoint_S0_002"
  Demux1/12 -> Bus Creator2/12  "Orientation_S0_002"
  Merge1/1 -> Demux1/1
  Bus Creator2/1 -> M01ObjInfo/1  "Obj2Info"
  obj_num/1 -> Relational Operator1/1
  Constant/1 -> Relational Operator1/2
  Relational Operator1/1 -> If Action Subsystem1/3(obj_trufal)
  Data Type Conversion1/1 -> If/1
  Data Type Conversion2/1 -> If/2
  Data Type Conversion3/1 -> If/3
  RemainderCnt/1 -> Data Type Conversion5/1, Subsystem1/2(RemainderCnt), Data Type Conversion3/1
  Subsystem1/1(Out) -> Add3/2
  Memory2/1 -> Subtract/2
  Subtract/1 -> Subsystem1/1(const)
  Memory3/1 -> Subsystem1/3(In)
  Data Type Conversion5/1 -> Subtract/1, Memory2/1

== system DFADAS2_SenFus_v1_201204RC_training_210115/Signal Input (Input)/Signal Input (50ms) (Input50)/Rear Left Radar(S0) Objects Information (RLRdr)/S0 Data Frame Read/Enabled Subsystem/M1ObjInfo1 ==
  msg : Inport
  MValue : Inport  Port=2
  RemainderCnt : Inport  Port=3
  obj_num : Inport  Port=4
  Add3 : Sum
  Bus Creator1 : BusCreator  Inputs=24
  Bus Creator2 : BusCreator  Inputs=24
  Constant : Constant  Value=3
  Data Type Conversion{,1..3} (4 alike) : DataTypeConversion  OutDataTypeStr=uint16
  Data Type Conversion5 : DataTypeConversion  OutDataTypeStr=int16
  Demux : Demux  Outputs=24
  Demux1 : Demux  Outputs=24
  If : If  NumInputs=3  IfExpression=u1 == 1  ElseIfExpressions=u2 == 0 & u3 == 1  ShowElse=off
  If Action Subsystem1 : Subsystem  TreatAsAtomicUnit=on
  If Action Subsystem2 : Subsystem  TreatAsAtomicUnit=on
  MValueSel : Constant
  Memory1 : Memory  InheritSampleTime=on
  Memory3 : Memory  InheritSampleTime=on
  Merge : Merge
  Merge1 : Merge
  Relational Operator : RelationalOperator  Operator===  OutDataTypeStr=boolean  RndMeth=Simplest
  Relational Operator1 : RelationalOperator  Operator=>  OutDataTypeStr=boolean  RndMeth=Simplest
  Scope1 : Scope
  Subsystem1 : Subsystem
  Subtract : Sum  Inputs=+-
  M10ObjInfo : Outport
  M11ObjInfo : Outport  Port=2
  wires:
  Bus Creator2/1 -> M11ObjInfo/1  "Obj4Info"
  Merge1/1 -> Demux1/1
  Demux1/12 -> Bus Creator2/12  "Orientation_S0_004"
  Demux1/17 -> Bus Creator2/17  "ReferencePoint_S0_004"
  Demux1/22 -> Bus Creator2/22  "YAccStd_S0_004"
  Demux1/23 -> Bus Creator2/23  "YPosStd_S0_004"
  Demux1/8 -> Bus Creator2/8  "XAcc_S0_004"
  Demux1/21 -> Bus Creator2/21  "XVelocityStd_S0_004"
  Demux1/19 -> Bus Creator2/19  "XAccStd_S0_004"
  Demux1/18 -> Bus Creator2/18  "Height_S0_004"
  Demux1/15 -> Bus Creator2/15  "ClassHighest_S0_004"
  Demux1/7 -> Bus Creator2/7  "YVelocity_S0_004"
  Demux1/14 -> Bus Creator2/14  "MovingState_S0_004"
  Demux1/20 -> Bus Creator2/20  "XPosStd_S0_004"
  Demux1/13 -> Bus Creator2/13  "ExistenceProb_S0_004"
  Demux1/9 -> Bus Creator2/9  "YAcc_S0_004"
  Demux1/24 -> Bus Creator2/24  "YVelocityStd_S0_004"
  Demux1/11 -> Bus Creator2/11  "Length_S0_004"
  Demux1/10 -> Bus Creator2/10  "Width_S0_004"
  Demux1/4 -> Bus Creator2/4  "XPos_S0_004"
  Demux1/16 -> Bus Creator2/16  "ClassHighestProb_S0_004"
  Demux1/5 -> Bus Creator2/5  "YPos_S0_004"
  Demux1/3 -> Bus Creator2/3  "ObjMeasured_S0_004"
  Demux1/2 -> Bus Creator2/2  "ObjInit_S0_004"
  Demux1/6 -> Bus Creator2/6  "XVelocity_S0_004"
  Demux1/1 -> Bus Creator2/1  "Id_S0_004"
  Demux/6 -> Bus Creator1/6  "XVelocity_S0_003"
  Demux/1 -> Scope1/1, Bus Creator1/1  "Id_S0_003"
  Demux/15 -> Bus Creator1/15  "ClassHighest_S0_003"
  Demux/11 -> Bus Creator1/11  "Length_S0_003"
  Demux/2 -> Bus Creator1/2  "ObjInit_S0_003"
  Demux/8 -> Bus Creator1/8  "XAcc_S0_003"
  Demux/19 -> Bus Creator1/19  "XAccStd_S0_003"
  Demux/4 -> Bus Creator1/4  "XPos_S0_003"
  Demux/21 -> Bus Creator1/21  "XVelocityStd_S0_003"
  Demux/16 -> Bus Creator1/16  "ClassHighestProb_S0_003"
  Demux/3 -> Bus Creator1/3  "ObjMeasured_S0_003"
  Demux/23 -> Bus Creator1/23  "YPosStd_S0_003"
  Demux/5 -> Bus Creator1/5  "YPos_S0_003"
  Demux/14 -> Bus Creator1/14  "MovingState_S0_003"
  Demux/9 -> Bus Creator1/9  "YAcc_S0_003"
  Demux/12 -> Bus Creator1/12  "Orientation_S0_003"
  Demux/18 -> Bus Creator1/18  "Height_S0_003"
  Demux/20 -> Bus Creator1/20  "XPosStd_S0_003"
  Demux/7 -> Bus Creator1/7  "YVelocity_S0_003"
  Demux/22 -> Bus Creator1/22  "YAccStd_S0_003"
  Demux/17 -> Bus Creator1/17  "ReferencePoint_S0_003"
  Demux/13 -> Bus Creator1/13  "ExistenceProb_S0_003"
  Demux/10 -> Bus Creator1/10  "Width_S0_003"
  Demux/24 -> Bus Creator1/24  "YVelocityStd_S0_003"
  Bus Creator1/1 -> M10ObjInfo/1  "Obj3Info"
  Merge/1 -> Demux/1
  Data Type Conversion3/1 -> If/3
  Data Type Conversion2/1 -> If/2
  Data Type Conversion1/1 -> If/1
  If Action Subsystem1/2(M11ObjInfo) -> Merge1/1
  If Action Subsystem2/2(ZeroObjInfo1) -> Merge1/2
  MValueSel/1 -> Relational Operator/1, If Action Subsystem1/2("MValueSel ")
  If Action Subsystem2/1(ZeroObjInfo0) -> Merge/2
  If Action Subsystem1/1(M10ObjInfo) -> Merge/1
  Relational Operator/1 -> Data Type Conversion1/1, Data Type Conversion/1
  If/2 -> If Action Subsystem2/Action
  If/1 -> If Action Subsystem1/Action
  Data Type Conversion/1 -> Add3/1
  Add3/1 -> Memory3/1, Data Type Conversion2/1  "MValueSim"
  MValue/1 -> Relational Operator/2
  msg/1 -> If Action Subsystem1/1(msg)
  Relational Operator1/1 -> If Action Subsystem1/3("0bj_d4 ")
  Constant/1 -> Relational Operator1/2
  obj_num/1 -> Relational Operator1/1
  Subsystem1/1(Out) -> Add3/2
  RemainderCnt/1 -> Data Type Conversion3/1, Data Type Conversion5/1
  Memory1/1 -> Subtract/2
  Subtract/1 -> Subsystem1/1(const)
  Data Type Conversion5/1 -> Subtract/1, Memory1/1
  Memory3/1 -> Subsystem1/3(In)

== system DFADAS2_SenFus_v1_201204RC_training_210115/Signal Input (Input)/Signal Input (50ms) (Input50)/Rear Left Radar(S0) Objects Information (RLRdr)/S0 Data Frame Read/Enabled Subsystem/M2ObjInfo ==
  msg : Inport
  MValue : Inport  Port=2
  RemainderCnt : Inport  Port=3
  obj_num : Inport  Port=4
  Add3 : Sum
  Bus Creator1 : BusCreator  Inputs=24
  Bus Creator2 : BusCreator  Inputs=24
  Constant : Constant  Value=5
  Data Type Conversion{,1..3} (4 alike) : DataTypeConversion  OutDataTypeStr=uint16
  Data Type Conversion5 : DataTypeConversion  OutDataTypeStr=int16
  Demux : Demux  Outputs=24
  Demux1 : Demux  Outputs=24
  If : If  NumInputs=3  IfExpression=u1 == 1  ElseIfExpressions=u2 == 0 & u3 == 1  ShowElse=off
  If Action Subsystem1 : Subsystem  TreatAsAtomicUnit=on
  If Action Subsystem2 : Subsystem  TreatAsAtomicUnit=on
  MValueSel : Constant  Value=2
  Memory1 : Memory  InheritSampleTime=on
  Memory3 : Memory  InheritSampleTime=on
  Merge : Merge
  Merge1 : Merge
  Relational Operator : RelationalOperator  Operator===  OutDataTypeStr=boolean  RndMeth=Simplest
  Relational Operator1 : RelationalOperator  Operator=>  OutDataTypeStr=boolean  RndMeth=Simplest
  Subsystem1 : Subsystem
  Subtract : Sum  Inputs=+-
  M20ObjInfo : Outport
  M21ObjInfo : Outport  Port=2
  wires:
  msg/1 -> If Action Subsystem1/1(msg)
  MValue/1 -> Relational Operator/2
  Subsystem1/1(Out) -> Add3/2
  Add3/1 -> Memory3/1, Data Type Conversion2/1  "MValueSim"
  Data Type Conversion/1 -> Add3/1
  If/1 -> If Action Subsystem1/Action
  If/2 -> If Action Subsystem2/Action
  Relational Operator/1 -> Data Type Conversion/1, Data Type Conversion1/1
  If Action Subsystem1/1(M20ObjInfo) -> Merge/1
  If Action Subsystem2/1(ZeroObjInfo0) -> Merge/2
  MValueSel/1 -> If Action Subsystem1/2("MValueSel "), Relational Operator/1
  If Action Subsystem2/2(ZeroObjInfo1) -> Merge1/2
  If Action Subsystem1/2(M21ObjInfo) -> Merge1/1
  Data Type Conversion1/1 -> If/1
  Data Type Conversion2/1 -> If/2
  Data Type Conversion3/1 -> If/3
  Merge/1 -> Demux/1
  Bus Creator1/1 -> M20ObjInfo/1  "Obj5Info"
  Demux/24 -> Bus Creator1/24  "YVelocityStd_S0_005"
  Demux/10 -> Bus Creator1/10  "Width_S0_005"
  Demux/13 -> Bus Creator1/13  "ExistenceProb_S0_005"
  Demux/17 -> Bus Creator1/17  "ReferencePoint_S0_005"
  Demux/22 -> Bus Creator1/22  "YAccStd_S0_005"
  Demux/7 -> Bus Creator1/7  "YVelocity_S0_005"
  Demux/20 -> Bus Creator1/20  "XPosStd_S0_005"
  Demux/18 -> Bus Creator1/18  "Height_S0_005"
  Demux/12 -> Bus Creator1/12  "Orientation_S0_005"
  Demux/9 -> Bus Creator1/9  "YAcc_S0_005"
  Demux/14 -> Bus Creator1/14  "MovingState_S0_005"
  Demux/5 -> Bus Creator1/5  "YPos_S0_005"
  Demux/23 -> Bus Creator1/23  "YPosStd_S0_005"
  Demux/3 -> Bus Creator1/3  "ObjMeasured_S0_005"
  Demux/16 -> Bus Creator1/16  "ClassHighestProb_S0_005"
  Demux/21 -> Bus Creator1/21  "XVelocityStd_S0_005"
  Demux/4 -> Bus Creator1/4  "XPos_S0_005"
  Demux/19 -> Bus Creator1/19  "XAccStd_S0_005"
  Demux/8 -> Bus Creator1/8  "XAcc_S0_005"
  Demux/2 -> Bus Creator1/2  "ObjInit_S0_005"
  Demux/11 -> Bus Creator1/11  "Length_S0_005"
  Demux/15 -> Bus Creator1/15  "ClassHighest_S0_005"
  Demux/1 -> Bus Creator1/1  "Id_S0_005"
  Demux/6 -> Bus Creator1/6  "XVelocity_S0_005"
  Demux1/1 -> Bus Creator2/1  "Id_S0_006"
  Demux1/6 -> Bus Creator2/6  "XVelocity_S0_006"
  Demux1/2 -> Bus Creator2/2  "ObjInit_S0_006"
  Demux1/3 -> Bus Creator2/3  "ObjMeasured_S0_006"
  Demux1/5 -> Bus Creator2/5  "YPos_S0_006"
  Demux1/16 -> Bus Creator2/16  "ClassHighestProb_S0_006"
  Demux1/4 -> Bus Creator2/4  "XPos_S0_006"
  Demux1/10 -> Bus Creator2/10  "Width_S0_006"
  Demux1/11 -> Bus Creator2/11  "Length_S0_006"
  Demux1/24 -> Bus Creator2/24  "YVelocityStd_S0_006"
  Demux1/9 -> Bus Creator2/9  "YAcc_S0_006"
  Demux1/13 -> Bus Creator2/13  "ExistenceProb_S0_006"
  Demux1/20 -> Bus Creator2/20  "XPosStd_S0_006"
  Demux1/14 -> Bus Creator2/14  "MovingState_S0_006"
  Demux1/7 -> Bus Creator2/7  "YVelocity_S0_006"
  Demux1/15 -> Bus Creator2/15  "ClassHighest_S0_006"
  Demux1/18 -> Bus Creator2/18  "Height_S0_006"
  Demux1/19 -> Bus Creator2/19  "XAccStd_S0_006"
  Demux1/21 -> Bus Creator2/21  "XVelocityStd_S0_006"
  Demux1/8 -> Bus Creator2/8  "XAcc_S0_006"
  Demux1/23 -> Bus Creator2/23  "YPosStd_S0_006"
  Demux1/22 -> Bus Creator2/22  "YAccStd_S0_006"
  Demux1/17 -> Bus Creator2/17  "ReferencePoint_S0_006"
  Demux1/12 -> Bus Creator2/12  "Orientation_S0_006"
  Merge1/1 -> Demux1/1
  Bus Creator2/1 -> M21ObjInfo/1  "Obj6Info"
  Relational Operator1/1 -> If Action Subsystem1/3("obj_count_trorfa ")
  Constant/1 -> Relational Operator1/2
  obj_num/1 -> Relational Operator1/1
  Subtract/1 -> Subsystem1/1(const)
  RemainderCnt/1 -> Data Type Conversion5/1, Data Type Conversion3/1
  Memory1/1 -> Subtract/2
  Data Type Conversion5/1 -> Subtract/1, Memory1/1
  Memory3/1 -> Subsystem1/3(In)
